simulink model "Hector_Simulation"  (R2023b)
settings: Solver=daessc  StartTime=0.0  StopTime=T-dt  FixedStep=0.001  MaxStep=1e-3  RelTol=1e-2
model workspace (MATLAB code in the model file):
  | %% World Plane
  | plane_x = 20;
  | plane_y = 2;
  | plane_z = 0.05;
  | 
  | %% motor
  | %A1
  | motor_com = [0, -0.02,0];
  | motor_com_mirror = [0, 0.02,0];
  | 
  | motor_I = [0.00048,0.00071,0.00048];
  | motor_mass = 0.605;
  | 
  | %% Body
  | % Inertial
  | body_com_x = 0.0;
  | body_com_y = 0.0;
  | body_com_z = -0.0;
  | body_mass = 5.75;
  | body_ixx = 44350*1e-6;
  | body_ixy = 0.0;
  | body_ixz = 0.0;
  | body_iyy = 53149*1e-6;
  | body_iyz = 0.0;
  | body_izz = 21390*1e-6;
  | 
  | %% Hip 1
  | % joint
  | hip1_offset_x =0.0;
  | hip1_offset_y = 0.047;
  | hip1_offset_z = 0.1265;
  | % hip1_max = 15;
  | % hip1_min = -15;
  | hip1_velocity_max = 21;
  | hip1_torque_max = 33.5;
  | % Inertial
  | hip1_com_x = 0.0268;
  | hip1_com_y = -0.00315;
  | hip1_com_z = -0.0272;
  | hip1_mass = 0.173;
  | hip1_ixx = 0.00022;
  | hip1_ixy = 0.0;
  | hip1_ixz = 0.0;
  | hip1_iyy = 0.00024;
  | hip1_iyz = 0.0;
  | hip1_izz = 0.00016;
  | 
  | %% Hip 2
  | % joint
  | hip2_offset_x =0.053;
  | hip2_offset_y = 0.0185;
  | hip2_offset_z = 0.071;
  | % hip2_max = 15;
  | % hip2_min = -15;
  | hip2_velocity_max = 21;
  | hip2_torque_max = 33.5;
  | % Inertial
  | hip2_com_x = -0.0308;
  | hip2_com_y = -0.00942;
  | hip2_com_z = 0.0;
  | hip2_mass = 0.0722;
  | hip2_ixx = 0.0000422;
  | hip2_ixy = 0.0;
  | hip2_ixz = 0.0;
  | hip2_iyy = 0.000120;
  | hip2_iyz = 0.0;
  | hip2_izz = 0.0000708;
  | 
  | %% Thigh
  | % joint
  | thigh_offset_x =-0.06;
  | thigh_offset_y = 0.004;
  | thigh_offset_z = 0.0;
  | % thigh_max = 130;
  | % thigh_min = -45;
  | thigh_velocity_max = 21;
  | thigh_torque_max = 33.5;
  | % Inertial
  | thigh_com_x = -0.00143;
  | thigh_com_y = -0.02106;
  | thigh_com_z = -0.06115;
  | thigh_mass = 0.397;
  | thigh_ixx = 0.00197;
  | thigh_ixy = 0.0;
  | thigh_ixz = 0.0;
  | thigh_iyy = 0.00218;
  | thigh_iyz = 0.0;
  | thigh_izz = 0.00033;
  | 
  | ankle_motor_offset_x = 0;
  | ankle_motor_offset_y = 0.039;
  | ankle_motor_offset_z = 0;
  | 
  | knee_motor_offset_x = 0;
  | knee_motor_offset_y = 0.039;
  | knee_motor_offset_z = -0.095;
  | 
  | %% Calf
  | % joint
  | calf_offset_x = 0.0;
  | calf_offset_y = 0.003;
  | calf_offset_z = -0.22;
  | % calf_max = 0;
  | % calf_min = -135;
  | % knee_max = 0;
  | % knee_min = -160;
  | calf_velocity_max = 14*1.5;
  | calf_torque_max = 51;
  | % Inertial
  | calf_com_x = 0.00165;
  | calf_com_y = -0.01117;
  | calf_com_z = -0.06438;
  | calf_mass = 0.136;
  | calf_ixx = 0.00071;
  | calf_ixy = 0.0;
  | calf_ixz = 0.0;
  | calf_iyy = 0.00072;
  | calf_iyz = 0.0;
  | calf_izz = 0.00002;
  | 
  | %% Toe
  | % joint
  | toe_offset_x = 0.0;
  | toe_offset_y = 0.011;
  | toe_offset_z = -0.22;
  | % toe_max = 60;
  | % toe_min = -60;
  | toe_velocity_max = 21;
  | toe_torque_max = 33.5;
  | % Inertial
  | toe_com_x = 0.00239;
  | toe_com_y = 0.00002;
  | toe_com_z = -0.02261;
  | toe_mass = 0.08425;
  | toe_ixx = 0.00001;
  | toe_ixy = 0.0;
  | toe_ixz = 0.0;
  | toe_iyy = 0.00011;
  | toe_iyz = 0.0;
  | toe_izz = 0.00011;
  | %% Contact
  | contact_front = 0.091;
  | contact_rear = -0.061;
  | contact_right = 0.026;
  | contact_left = 0.01;
  | contact_z = 0.039;
  | 
  | %%
  | %dorito
  | dorito_offset_x = 0;
  | dorito_offset_y = 0.012;
  | dorito_offset_z = 0;
  | 
  | dorito_lower_connection = [0.034 0 -0.044];
  | dorito_upper_connection = [0.034 0 0.021];
  | 
  | linkage_mass = 0.051;
  | linkage_com = [0 0 -0.11];
  | linkage_I = [0.00001 0.00002 0.00002];
  | 
  | % linkage_mass = 0.00001;
  | % linkage_com = [0 0 -0.11];
  | % linkage_I = [0.00000001 0.00000001 0.00000001];
  | 
  | misc_mass = 0.0001;
  | %% Arms
  | shoulder_com_x = 0;
  | shoulder_com_y = 0;
  | shoulder_com_z = 0;
  | shoulder_mass = 0.835;
  | % shoulder_mass = 0.05;
  | shoulder_ixx = 920*1e-6;
  | shoulder_ixy = 0.0;
  | shoulder_ixz = 0.0;
  | shoulder_iyy = 270*1e-6;
  | shoulder_iyz = 0.0;
  | shoulder_izz = 499*1e-6;
  | 
  | upperarm_com_x = 0;
  | upperarm_com_y = 0;
  | upperarm_com_z = 0;
  | upperarm_mass = 1.35;
  | % upperarm_mass = 0.05;
  | upperarm_ixx = 1200*1e-6;
  | upperarm_ixy = 0.0;
  | upperarm_ixz = 0.0;
  | upperarm_iyy = 1170*1e-6;
  | upperarm_iyz = 0.0;
  | upperarm_izz = 729*1e-6;
  | 
  | forearm_com_x = 0;
  | forearm_com_y = 0;
  | forearm_com_z = -0.10;
  | forearm_mass = 0.53;
  | % forearm_mass = 0.03;
  | forearm_ixx = 427*1e-6;
  | forearm_ixy = 0.0;
  | forearm_ixz = 0.0;
  | forearm_iyy = 466*1e-6;
  | forearm_iyz = 0.0;
  | forearm_izz = 72*1e-6;
undefined symbols (not defined in the file): ankle_damping, AssignMPCStage, body_v0, body_z0, control, dt, joint_damping, option, Q_TO, sigbuilder_block, X, Y, Z
libraries: sm_lib x141, nesl_utility x79, simulink x1
(part 6 of 6)

== system Hector_Simulation/Hector/Right Leg/Package Measurements 3D/Extract Measurements ==
  meas : Inport
  Bus Selector : BusSelector  OutputSignals=angle,speed,torque
  angle : Outport  VectorParamsAs1DForOutWhenUnconnected=off
  speed : Outport  Port=2  VectorParamsAs1DForOutWhenUnconnected=off
  torque : Outport  Port=3  VectorParamsAs1DForOutWhenUnconnected=off
  wires:
  Bus Selector/3 -> torque/1  "<torque>"
  meas/1 -> Bus Selector/1
  Bus Selector/1 -> angle/1  "<angle>"
  Bus Selector/2 -> speed/1  "<speed>"

== system Hector_Simulation/Hector/Right Leg/Package Measurements 3D/Extract Measurements1 ==
  meas : Inport
  Bus Selector : BusSelector  OutputSignals=angle,speed,torque
  angle : Outport  VectorParamsAs1DForOutWhenUnconnected=off
  speed : Outport  Port=2  VectorParamsAs1DForOutWhenUnconnected=off
  torque : Outport  Port=3  VectorParamsAs1DForOutWhenUnconnected=off
  wires:
  Bus Selector/2 -> speed/1  "<speed>"
  Bus Selector/1 -> angle/1  "<angle>"
  meas/1 -> Bus Selector/1
  Bus Selector/3 -> torque/1  "<torque>"

== system Hector_Simulation/Hector/Right Leg/Package Measurements 3D/Extract Measurements2 ==
  meas : Inport
  Bus Selector : BusSelector  OutputSignals=angle,speed,torque
  angle : Outport  VectorParamsAs1DForOutWhenUnconnected=off
  speed : Outport  Port=2  VectorParamsAs1DForOutWhenUnconnected=off
  torque : Outport  Port=3  VectorParamsAs1DForOutWhenUnconnected=off
  wires:
  Bus Selector/3 -> torque/1  "<torque>"
  meas/1 -> Bus Selector/1
  Bus Selector/1 -> angle/1  "<angle>"
  Bus Selector/2 -> speed/1  "<speed>"

== system Hector_Simulation/Hector/Right Leg/Package Measurements 3D/Extract Measurements3 ==
  meas : Inport
  Bus Selector : BusSelector  OutputSignals=angle,speed,torque
  angle : Outport  VectorParamsAs1DForOutWhenUnconnected=off
  speed : Outport  Port=2  VectorParamsAs1DForOutWhenUnconnected=off
  torque : Outport  Port=3  VectorParamsAs1DForOutWhenUnconnected=off
  wires:
  Bus Selector/2 -> speed/1  "<speed>"
  Bus Selector/1 -> angle/1  "<angle>"
  meas/1 -> Bus Selector/1
  Bus Selector/3 -> torque/1  "<torque>"

== system Hector_Simulation/Hector/Right Leg/Package Measurements 3D/Extract Measurements4 ==
  meas : Inport
  Bus Selector : BusSelector  OutputSignals=angle,speed,torque
  angle : Outport  VectorParamsAs1DForOutWhenUnconnected=off
  speed : Outport  Port=2  VectorParamsAs1DForOutWhenUnconnected=off
  torque : Outport  Port=3  VectorParamsAs1DForOutWhenUnconnected=off
  wires:
  Bus Selector/3 -> torque/1  "<torque>"
  meas/1 -> Bus Selector/1
  Bus Selector/1 -> angle/1  "<angle>"
  Bus Selector/2 -> speed/1  "<speed>"

== system Hector_Simulation/Hector/Right Leg/Thigh/Hip Pitch Joint ==
  Joint : Inport
  Bus Creator : BusCreator  Inputs=3
  Hip Pitch : sm_lib/Joints/Revolute Joint  JointMode=Normal  SenseConstraintForce=off  SenseConstraintForceX=off  SenseConstraintForceY=off  SenseConstraintForceZ=off  SenseConstraintTorque=off  SenseConstraintTorqueX=off  SenseConstraintTorqueY=off  SenseConstraintTorqueZ=off  SenseTotalForce=off  SenseTotalForceX=off  SenseTotalForceY=off  SenseTotalForceZ=off  SenseTotalTorque=off  SenseTotalTorqueX=off  SenseTotalTorqueY=off  SenseTotalTorqueZ=off  CompositeWrenchDir=FollowerOnBase  CompositeWrenchFrame=BaseFrame  EquilibriumPosition=0  EquilibriumPositionUnits=deg  SpringStiffness=0  SpringStiffnessUnits=N*m/deg  DampingCoefficient=joint_damping/2  DampingCoefficientUnits=N*m/(rad/s)  TorqueActuationMode=InputTorque  MotionActuationMode=ComputedMotion  SensePosition=on  SenseVelocity=on  SenseAcceleration=off  SenseTorqueForce=off  SenseLowerLimitTorqueForce=off  SenseUpperLimitTorqueForce=off  LowerLimitSpecify=on  LowerLimitBound=thigh_min  LowerLimitBoundUnits=deg  LowerLimitStiffness=limit_stiffness  LowerLimitStiffnessUnits=N*m/deg  LowerLimitDamping=limit_damping  LowerLimitDampingUnits=N*m/(deg/s)  LowerLimitTransitionRegionWidth=0.1  LowerLimitTransitionRegionWidthUnits=deg  UpperLimitSpecify=on  UpperLimitBound=thigh_max  UpperLimitBoundUnits=deg  UpperLimitStiffness=limit_stiffness  UpperLimitStiffnessUnits=N*m/deg  UpperLimitDamping=limit_damping  UpperLimitDampingUnits=N*m/(deg/s)  UpperLimitTransitionRegionWidth=0.1  UpperLimitTransitionRegionWidthUnits=deg  PositionTargetSpecify=on  PositionTargetPriority=High  PositionTargetValue=thigh_q0  PositionTargetValueUnits=deg  VelocityTargetSpecify=off  VelocityTargetPriority=High  VelocityTargetValue=0  VelocityTargetValueUnits=deg/s
  PS-Simulink Converter : nesl_utility/PS-Simulink Converter  PhysicalDomain=network_engine_domain  SubClassName=ps_output  LeftPortType=input  RightPortType=output  PseudoPeriodic=off  Frequencies=[]  VectorFormat=1-D array  Unit=rad  AffineConversion=off
  PS-Simulink Converter1 : nesl_utility/PS-Simulink Converter  PhysicalDomain=network_engine_domain  SubClassName=ps_output  LeftPortType=input  RightPortType=output  PseudoPeriodic=off  Frequencies=[]  VectorFormat=1-D array  Unit=rad/s  AffineConversion=off
  Simulink-PS Converter : nesl_utility/Simulink-PS Converter  PhysicalDomain=network_engine_domain  SubClassName=ps_input  LeftPortType=input  RightPortType=output  PseudoPeriodic=off  Frequencies=[]  NoiseDistribution=none  NoiseParameters=[]  Unit=1  AffineConversion=off  FilteringAndDerivatives=provide  SimscapeFilterOrder=1  InputFilterTimeConstant=0.001  UdotUserProvided=0
  B : PMIOPort  Side=Left
  F : PMIOPort  Port=2  Side=Right
  Sensor : Outport
  wires:
  PS-Simulink Converter/1 -> Bus Creator/1  "angle"
  Joint/1 -> Bus Creator/3, Simulink-PS Converter/1  "torque"
  Bus Creator/1 -> Sensor/1
  PS-Simulink Converter1/1 -> Bus Creator/2  "speed"
  connections:
  Hip Pitch/RConn2 -- PS-Simulink Converter/LConn1
  Simulink-PS Converter/RConn1 -- Hip Pitch/LConn2
  Hip Pitch/LConn1 -- B/RConn1
  Hip Pitch/RConn3 -- PS-Simulink Converter1/LConn1
  F/RConn1 -- Hip Pitch/RConn1

== system Hector_Simulation/Hector/Right Leg/calf/Knee Joint ==
  Joint : Inport
  Bus Creator : BusCreator  Inputs=3
  Knee Joint : sm_lib/Joints/Revolute Joint  JointMode=Normal  SenseConstraintForce=off  SenseConstraintForceX=off  SenseConstraintForceY=off  SenseConstraintForceZ=off  SenseConstraintTorque=off  SenseConstraintTorqueX=off  SenseConstraintTorqueY=off  SenseConstraintTorqueZ=off  SenseTotalForce=off  SenseTotalForceX=off  SenseTotalForceY=off  SenseTotalForceZ=off  SenseTotalTorque=off  SenseTotalTorqueX=off  SenseTotalTorqueY=off  SenseTotalTorqueZ=off  CompositeWrenchDir=FollowerOnBase  CompositeWrenchFrame=BaseFrame  EquilibriumPosition=0  EquilibriumPositionUnits=deg  SpringStiffness=0  SpringStiffnessUnits=N*m/deg  DampingCoefficient=joint_damping/2  DampingCoefficientUnits=N*m/(rad/s)  TorqueActuationMode=InputTorque  MotionActuationMode=ComputedMotion  SensePosition=on  SenseVelocity=on  SenseAcceleration=off  SenseTorqueForce=off  SenseLowerLimitTorqueForce=off  SenseUpperLimitTorqueForce=off  LowerLimitSpecify=on  LowerLimitBound=knee_min  LowerLimitBoundUnits=deg  LowerLimitStiffness=limit_stiffness  LowerLimitStiffnessUnits=N*m/deg  LowerLimitDamping=limit_damping  LowerLimitDampingUnits=N*m/(deg/s)  LowerLimitTransitionRegionWidth=0.1  LowerLimitTransitionRegionWidthUnits=deg  UpperLimitSpecify=on  UpperLimitBound=knee_max  UpperLimitBoundUnits=deg  UpperLimitStiffness=limit_stiffness  UpperLimitStiffnessUnits=N*m/deg  UpperLimitDamping=limit_damping  UpperLimitDampingUnits=N*m/(deg/s)  UpperLimitTransitionRegionWidth=0.1  UpperLimitTransitionRegionWidthUnits=deg  PositionTargetSpecify=on  PositionTargetPriority=High  PositionTargetValue=calf_q0  PositionTargetValueUnits=deg  VelocityTargetSpecify=off  VelocityTargetPriority=High  VelocityTargetValue=0  VelocityTargetValueUnits=deg/s
  PS-Simulink Converter : nesl_utility/PS-Simulink Converter  PhysicalDomain=network_engine_domain  SubClassName=ps_output  LeftPortType=input  RightPortType=output  PseudoPeriodic=off  Frequencies=[]  VectorFormat=1-D array  Unit=rad/s  AffineConversion=off
  PS-Simulink Converter1 : nesl_utility/PS-Simulink Converter  PhysicalDomain=network_engine_domain  SubClassName=ps_output  LeftPortType=input  RightPortType=output  PseudoPeriodic=off  Frequencies=[]  VectorFormat=1-D array  Unit=rad  AffineConversion=off
  Simulink-PS Converter : nesl_utility/Simulink-PS Converter  PhysicalDomain=network_engine_domain  SubClassName=ps_input  LeftPortType=input  RightPortType=output  PseudoPeriodic=off  Frequencies=[]  NoiseDistribution=none  NoiseParameters=[]  Unit=1  AffineConversion=off  FilteringAndDerivatives=provide  SimscapeFilterOrder=1  InputFilterTimeConstant=0.001  UdotUserProvided=0
  B : PMIOPort  Side=Left
  F : PMIOPort  Port=2  Side=Right
  Sensor : Outport
  wires:
  PS-Simulink Converter1/1 -> Bus Creator/1  "angle"
  Bus Creator/1 -> Sensor/1
  Joint/1 -> Bus Creator/3, Simulink-PS Converter/1  "torque"
  PS-Simulink Converter/1 -> Bus Creator/2  "speed"
  connections:
  Knee Joint/RConn3 -- PS-Simulink Converter/LConn1
  Knee Joint/RConn1 -- F/RConn1
  Knee Joint/RConn2 -- PS-Simulink Converter1/LConn1
  Simulink-PS Converter/RConn1 -- Knee Joint/LConn2
  Knee Joint/LConn1 -- B/RConn1

== system Hector_Simulation/Hector/Right Leg/foot/Ankle Joint ==
  input : Inport
  Ankle Joint : sm_lib/Joints/Revolute Joint  JointMode=Normal  SenseConstraintForce=off  SenseConstraintForceX=off  SenseConstraintForceY=off  SenseConstraintForceZ=off  SenseConstraintTorque=off  SenseConstraintTorqueX=off  SenseConstraintTorqueY=off  SenseConstraintTorqueZ=off  SenseTotalForce=off  SenseTotalForceX=off  SenseTotalForceY=off  SenseTotalForceZ=off  SenseTotalTorque=off  SenseTotalTorqueX=off  SenseTotalTorqueY=off  SenseTotalTorqueZ=off  CompositeWrenchDir=FollowerOnBase  CompositeWrenchFrame=BaseFrame  EquilibriumPosition=0  EquilibriumPositionUnits=deg  SpringStiffness=0  SpringStiffnessUnits=N*m/deg  DampingCoefficient=ankle_damping/2  DampingCoefficientUnits=N*m/(rad/s)  TorqueActuationMode=InputTorque  MotionActuationMode=ComputedMotion  SensePosition=on  SenseVelocity=on  SenseAcceleration=off  SenseTorqueForce=off  SenseLowerLimitTorqueForce=off  SenseUpperLimitTorqueForce=off  LowerLimitSpecify=on  LowerLimitBound=ankle_min  LowerLimitBoundUnits=deg  LowerLimitStiffness=limit_stiffness  LowerLimitStiffnessUnits=N*m/deg  LowerLimitDamping=limit_damping  LowerLimitDampingUnits=N*m/(deg/s)  LowerLimitTransitionRegionWidth=0.1  LowerLimitTransitionRegionWidthUnits=deg  UpperLimitSpecify=on  UpperLimitBound=ankle_max  UpperLimitBoundUnits=deg  UpperLimitStiffness=limit_stiffness  UpperLimitStiffnessUnits=N*m/deg  UpperLimitDamping=limit_damping  UpperLimitDampingUnits=N*m/(deg/s)  UpperLimitTransitionRegionWidth=0.1  UpperLimitTransitionRegionWidthUnits=deg  PositionTargetSpecify=on  PositionTargetPriority=High  PositionTargetValue=toe_q0  PositionTargetValueUnits=deg  VelocityTargetSpecify=off  VelocityTargetPriority=High  VelocityTargetValue=0  VelocityTargetValueUnits=deg/s
  Bus Creator1 : BusCreator  Inputs=3
  PS-Simulink Converter : nesl_utility/PS-Simulink Converter  PhysicalDomain=network_engine_domain  SubClassName=ps_output  LeftPortType=input  RightPortType=output  PseudoPeriodic=off  Frequencies=[]  VectorFormat=inherit  Unit=inherit  AffineConversion=off
  PS-Simulink Converter1 : nesl_utility/PS-Simulink Converter  PhysicalDomain=network_engine_domain  SubClassName=ps_output  LeftPortType=input  RightPortType=output  PseudoPeriodic=off  Frequencies=[]  VectorFormat=inherit  Unit=inherit  AffineConversion=off
  Simulink-PS Converter : nesl_utility/Simulink-PS Converter  PhysicalDomain=network_engine_domain  SubClassName=ps_input  LeftPortType=input  RightPortType=output  PseudoPeriodic=off  Frequencies=[]  NoiseDistribution=none  NoiseParameters=[]  Unit=1  AffineConversion=off  FilteringAndDerivatives=provide  SimscapeFilterOrder=1  InputFilterTimeConstant=0.001  UdotUserProvided=0
  B : PMIOPort  Side=Left
  F : PMIOPort  Port=2  Side=Right
  sensor : Outport
  wires:
  PS-Simulink Converter1/1 -> Bus Creator1/2  "speed"
  PS-Simulink Converter/1 -> Bus Creator1/1  "angle"
  Bus Creator1/1 -> sensor/1
  input/1 -> Bus Creator1/3, Simulink-PS Converter/1  "torque"
  connections:
  Ankle Joint/LConn1 -- B/RConn1
  F/RConn1 -- Ankle Joint/RConn1
  Ankle Joint/RConn3 -- PS-Simulink Converter1/LConn1
  Ankle Joint/RConn2 -- PS-Simulink Converter/LConn1
  Simulink-PS Converter/RConn1 -- Ankle Joint/LConn2

== matlab function Hector_Simulation/Controllers/MATLAB Function ==
  data: t input; tauOut output; Q input; tau input; dt_sim input; q input; dq input; q_diff output; dq_diff output
function [tauOut, q_diff, dq_diff] = jointPD_Hector2D(t, Q, tau,dt_sim, q, dq)

Kp = 100;
Kd = 0.25;
N_input = length(tau(1,:));

%find index of nearest TO timestep
k = round(t/dt_sim)+1;

%upper bound of index is max length of simulation
k = min(k,N_input);

%%
t_active = 0;
%if prior to simulation start, zero out torques
if t <= t_active
    tauOut = zeros(10,1);
    q_diff = zeros(9, 1);
    dq_diff = zeros(9, 1);
else

    tau_hip_yaw_des_k = 0;
    q_hip_yaw_des_k = 0;
    dq_hip_yaw_des_k = 0;

    tau_hip_roll_des_k = 0;
    q_hip_roll_des_k = 0;
    dq_hip_roll_des_k = 0;

    tau_hip_pitch_des_k = tau(1,k)/2;
    q_hip_pitch_des_k = Q(4,k);
    
    tau_knee_des_k = tau(2,k)/2;
    q_knee_des_k = Q(5,k);

    tau_ankle_des_k = tau(3,k)/2;
    q_ankle_des_k = Q(6,k);
    
    if k == 1 || k == N_input
        dq_hip_pitch_des_k = 0; 
        dq_knee_des_k = 0;
        dq_ankle_des_k = 0;
    else
        dq_hip_pitch_des_k = (Q(4,k+1)-Q(4,k-1))/(2*dt_sim);  
        dq_knee_des_k = (Q(5,k+1)-Q(5,k-1))/(2*dt_sim); 
        dq_ankle_des_k = (Q(6,k+1)-Q(6,k-1))/(2*dt_sim); 
    end

    qR = q(1:5);
    qL = q(6:10);
    dqR = dq(1:5);
    dqL = dq(6:10);

    tau_hip_yawR = tau_hip_yaw_des_k+Kp*(q_hip_yaw_des_k-qR(1))+Kd*(dq_hip_yaw_des_k-dqR(1));
    tau_hip_rollR = tau_hip_roll_des_k+Kp*(q_hip_roll_des_k-qR(2))+Kd*(dq_hip_roll_des_k-dqR(2));
    tau_hip_pitchR = tau_hip_pitch_des_k+Kp*(q_hip_pitch_des_k-qR(3))+Kd*(dq_hip_pitch_des_k-dqR(3));
    tau_kneeR = tau_knee_des_k+Kp*(q_knee_des_k-qR(4))+Kd*(dq_knee_des_k-dqR(4));
    tau_ankleR = tau_ankle_des_k+Kp*(q_ankle_des_k-qR(5))+Kd*(dq_ankle_des_k-dqR(5));

    tau_hip_yawL = tau_hip_yaw_des_k+Kp*(q_hip_yaw_des_k-qL(1))+Kd*(dq_hip_yaw_des_k-dqL(1));
    tau_hip_rollL = tau_hip_roll_des_k+Kp*(q_hip_roll_des_k-qL(2))+Kd*(dq_hip_roll_des_k-dqL(2));
    tau_hip_pitchL = tau_hip_pitch_des_k+Kp*(q_hip_pitch_des_k-qL(3))+Kd*(dq_hip_pitch_des_k-dqL(3));
    tau_kneeL = tau_knee_des_k+Kp*(q_knee_des_k-qL(4))+Kd*(dq_knee_des_k-dqL(4));
    tau_ankleL = tau_ankle_des_k+Kp*(q_ankle_des_k-qL(5))+Kd*(dq_ankle_des_k-dqL(5));

    tauOut = [tau_hip_yawR; tau_hip_rollR; tau_hip_pitchR; tau_kneeR; tau_ankleR; tau_hip_yawL; tau_hip_rollL; tau_hip_pitchL; tau_kneeL; tau_ankleL];

    q_diff = [q_hip_pitch_des_k; qR(3); qL(3); q_knee_des_k; qR(4); qL(4); q_ankle_des_k; qR(5); qL(5)];
    dq_diff = [dq_hip_pitch_des_k; dqR(3); dqL(3); dq_knee_des_k; dqR(4); dqL(4); dq_ankle_des_k; dqR(5); dqL(5)];
end
